simulink model "l10_final"  (R2021b)
settings: Solver=VariableStepAuto  StartTime=0.0  StopTime=100  RelTol=1e-3
values from neighbouring files (symbols this model uses):
  g = 9.8    [exp10.m]
  K = 1    [exp10.m]
  l = 1    [exp10.m]
  mc = 10    [exp10.m]
  ml = 10    [exp10.m]
libraries: dspsrcs4 x1, simulink x1
settings Model: Creator=HP  LastModifiedBy=tushxr16

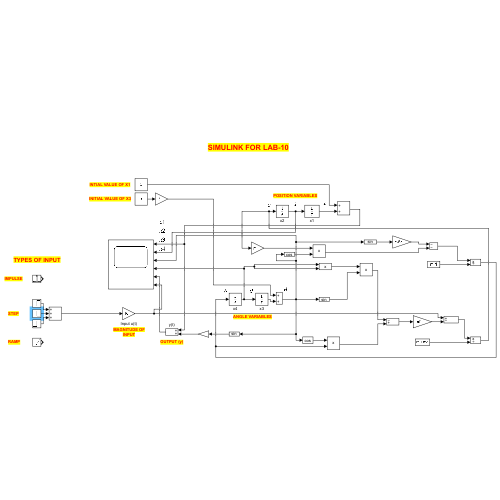
[thumbnail: Simulink's stored preview of the top-level diagram]
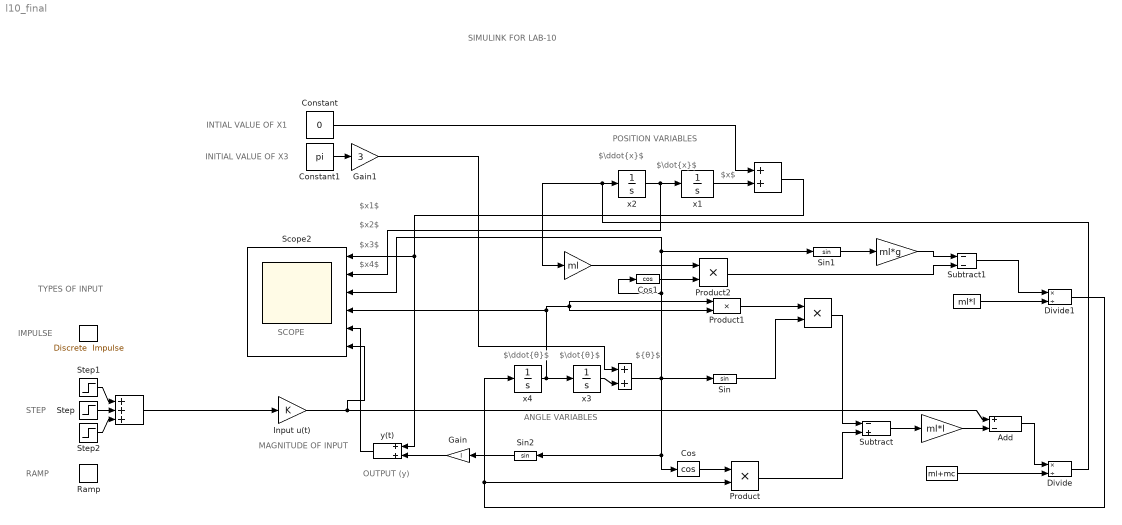
== system l10_final ==
  note: SCOPE
  note: $x2$
  note: $x1$
  note: $\dot{x}$
  note: $\ddot{x}$
  note: $\ddot{θ}$
  note: $\dot{θ}$
  note: ${θ}$
  note: $x3$
  note: $x4$
  note: $x$
  note: MAGNITUDE OF
      | INPUT
  note: OUTPUT (y)
  note: POSITION VARIABLES
  note: ANGLE VARIABLES
  note: IMPULSE
  note: STEP
  note: RAMP
  note: INITIAL VALUE OF X3
  note: INTIAL VALUE OF X1
  note: SIMULINK FOR LAB-10
  note: TYPES OF INPUT
  " " : dspsrcs4/Discrete  Impulse  Delay=0  SampleTime=1  FrameSample=1  OutputFrames=off  dataType=double  isSigned=on  wordLen=16  udDataType=sfix(16)  fracBitsMode=Best precision  numFracBits=15  OutDataTypeStr=double  LastOutDataTypeStr=double
  "  " : Sum  Inputs=+++
  "        " : Constant  Value=ml+mc
  "             " : Gain  Gain=ml*l
  "                      " : Sum
  "                       " : Gain  Gain=ml
  "                           " : Constant  Value=ml*l
  "                                " : Sum
  "                                                 " : Product
  "                                                  " : Gain  Gain=ml*g
  Add : Sum  Inputs=+-
  Constant : Constant  Value=0
  Constant1 : Constant  Value=pi
  Cos : Trigonometry  Operator=cos
  Cos1 : Trigonometry  Operator=cos
  Divide : Product  Inputs=*/
  Divide1 : Product  Inputs=*/
  Gain : Gain  Gain=l
  Gain1 : Gain  Gain=3
  Input u(t) : Gain  Gain=K
  Product : Product
  Product1 : Product
  Product2 : Product
  Ramp : simulink/Sources/Ramp  slope=1  start=0  InitialOutput=0
  Scope2 : Scope  NumInputPorts=6
  Sin : Trigonometry
  Sin1 : Trigonometry
  Sin2 : Trigonometry
  Step : Step  Time=t  After=-2  SampleTime=0
  Step1 : Step  Time=0  SampleTime=0
  Step2 : Step  Time=2*t  SampleTime=0
  Subtract : Sum  Inputs=-+
  Subtract1 : Sum  Inputs=--
  x{1..4} (4 alike) : Integrator
  y(t) : Sum
  wires:
  x2/1 -> Scope2/2, x1/1
  Divide/1 -> x2/1, "                       "/1
  Divide1/1 -> x4/1, Product/2
  x4/1 -> Product1/2, Product1/1, Scope2/4, x3/1
  Cos/1 -> Product/1
  Subtract/1 -> "             "/1
  "             "/1 -> Add/2
  Add/1 -> Divide/1
  "        "/1 -> Divide/2
  Cos1/1 -> Product2/2
  "                       "/1 -> Product2/1
  Sin1/1 -> "                                                  "/1
  "                                                  "/1 -> Subtract1/1
  Product2/1 -> Subtract1/2
  Subtract1/1 -> Divide1/1
  "                           "/1 -> Divide1/2
  Product1/1 -> "                                                 "/1
  Sin/1 -> "                                                 "/2
  "                                                 "/1 -> Subtract/1
  Product/1 -> Subtract/2
  Sin2/1 -> Gain/1
  Gain/1 -> y(t)/2
  y(t)/1 -> Scope2/5
  Input u(t)/1 -> Add/1, Scope2/6
  Step1/1 -> "  "/1
  "                                "/1 -> Scope2/3, Sin1/1, Cos1/1, Sin/1, Cos/1, Sin2/1
  x3/1 -> "                                "/2
  x1/1 -> "                      "/2
  Constant/1 -> "                      "/1
  "                      "/1 -> Scope2/1, y(t)/1
  Constant1/1 -> Gain1/1
  Gain1/1 -> "                                "/1
  "  "/1 -> Input u(t)/1
  Step/1 -> "  "/2
  Step2/1 -> "  "/3
